simulink model "openMHA_test_ar_filter_gaintable"  (R2020a)
settings: Solver=VariableStepAuto  StartTime=0.0  StopTime=stop_time  RelTol=1e-3
InitFcn:
  | test_ar_filter_gaintable_init
StopFcn:
  | test_ar_filter_gaintable_stop
values from neighbouring files (symbols this model uses):
  c1_a = exp( -1.0/(tau_a * fs) )    [test_FFT_to_gain_init.m]    (also in test_ar_filter_gaintable_init.m; test_ar_filter_init.m; test_db_ar_gaintable_init.m)
  c1_r = exp( -1.0/(tau_r * fs) )    [test_FFT_to_gain_init.m]    (also in test_ar_filter_gaintable_init.m; test_ar_filter_init.m; test_db_ar_gaintable_init.m)
  c2_a = 1.0 - c1_a    [test_FFT_to_gain_init.m]    (also in test_ar_filter_gaintable_init.m; test_ar_filter_init.m; test_db_ar_gaintable_init.m)
  c2_r = 1.0 - c1_r    [test_FFT_to_gain_init.m]    (also in test_ar_filter_gaintable_init.m; test_ar_filter_init.m; test_db_ar_gaintable_init.m)
  table_length = length(gtdata)    [calculate_gaintable.m]    (also in test_FFT_to_gain_init.m; test_ar_filter_gaintable_init.m; test_db_ar_gaintable_init.m; test_db_lookup_gain_fpga_init.m)
  X_high = 93    [test_FFT_to_gain_init.m]    (also in test_ar_filter_gaintable_init.m = 95; test_db_ar_gaintable_init.m; test_db_lookup_gain_fpga_init.m = 95; test_db_lookup_init.m = 95)
libraries: simulink x4, FPGA_Open_Speech_Tools x2, dspsrcs4 x1
settings Model: PacingRate=200  Creator=t96f346  LastModifiedBy=t96f346

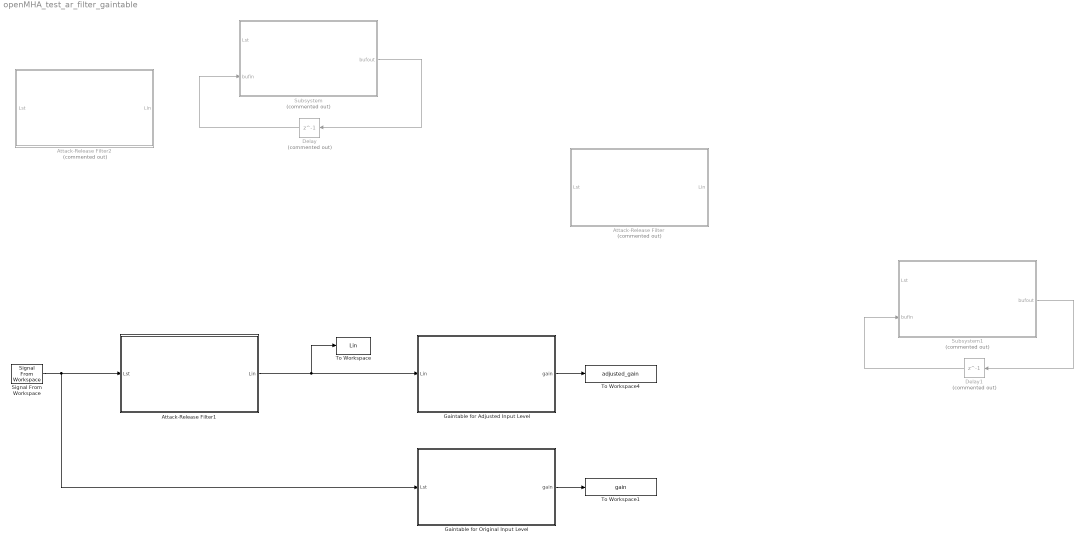
== system openMHA_test_ar_filter_gaintable ==
  Attack-Release Filter : Subsystem  Commented=on
  Attack-Release Filter1 : Subsystem
  Attack-Release Filter2 : Subsystem  Commented=on
  Delay : Delay  Commented=on  DelayLength=1  InitialCondition=65
  Delay1 : Delay  Commented=on  DelayLength=1  InitialCondition=65
  Gaintable for Adjusted Input Level : Subsystem
  Gaintable for Original Input Level : Subsystem
  Signal From Workspace : dspsrcs4/Signal From Workspace  X=Lst  Ts=1  nsamps=1  OutputAfterFinalValue=Setting to zero  ignoreOrWarnInputAndFrameLengths=off  OutputFrames=off
  Subsystem : Subsystem  Commented=on
  Subsystem1 : Subsystem  Commented=on
  To Workspace : ToWorkspace  VariableName=Lin  SampleTime=-1
      settings: Save2DSignal=2-D array (concatenate along first dimension)
  To Workspace1 : ToWorkspace  VariableName=gain  SampleTime=-1
      settings: Save2DSignal=2-D array (concatenate along first dimension)
  To Workspace4 : ToWorkspace  VariableName=adjusted_gain  SampleTime=-1
      settings: Save2DSignal=2-D array (concatenate along first dimension)
  wires:
  Delay/1 -> Subsystem/2(bufin)
  Subsystem/1(bufout) -> Delay/1
  Attack-Release Filter1/1(Lin) -> To Workspace/1, Gaintable for Adjusted Input Level/1(Lin)
  Gaintable for Adjusted Input Level/1(gain) -> To Workspace4/1
  Gaintable for Original Input Level/1(gain) -> To Workspace1/1
  Signal From Workspace/1 -> Attack-Release Filter1/1(Lst), Gaintable for Original Input Level/1(Lst)
  Delay1/1 -> Subsystem1/2(bufin)
  Subsystem1/1(bufout) -> Delay1/1

== system openMHA_test_ar_filter_gaintable/Attack-Release Filter ==
  Lst : Inport
  Delay2 : Delay  DelayLength=1  InitialCondition=65
  Release Filter : Subsystem  TreatAsAtomicUnit=on
  Lin : Outport  VectorParamsAs1DForOutWhenUnconnected=off
  wires:
  Release Filter/1(bufout) -> Lin/1, Delay2/1
  Lst/1 -> Release Filter/1(La)
  Delay2/1 -> Release Filter/2(bufin)

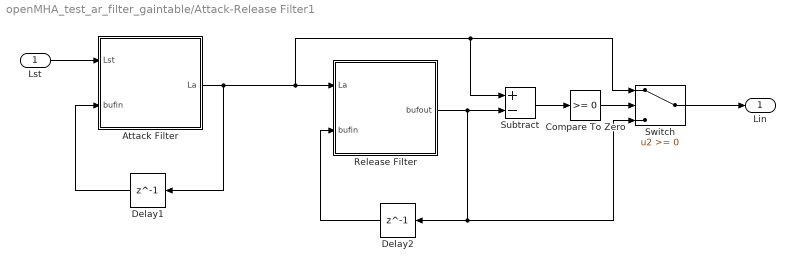
== system openMHA_test_ar_filter_gaintable/Attack-Release Filter1 ==
  Lst : Inport
  Attack Filter : Subsystem  TreatAsAtomicUnit=on
  Compare To Zero : simulink/Logic and Bit Operations/Compare To Zero  relop=>=  OutDataTypeStr=boolean
  Delay1 : Delay  DelayLength=1  InitialCondition=65
  Delay2 : Delay  DelayLength=1  InitialCondition=65
  Release Filter : Subsystem  TreatAsAtomicUnit=on
  Subtract : Sum  Inputs=+-  OutDataTypeStr=Inherit: Same as accumulator
  Switch : Switch
  Lin : Outport  VectorParamsAs1DForOutWhenUnconnected=off
  wires:
  Lst/1 -> Attack Filter/1(Lst)
  Delay2/1 -> Release Filter/2(bufin)
  Delay1/1 -> Attack Filter/2(bufin)
  Release Filter/1(bufout) -> Switch/3, Delay2/1, Subtract/2
  Switch/1 -> Lin/1
  Compare To Zero/1 -> Switch/2
  Attack Filter/1(La) -> Subtract/1, Switch/1, Release Filter/1(La), Delay1/1
  Subtract/1 -> Compare To Zero/1

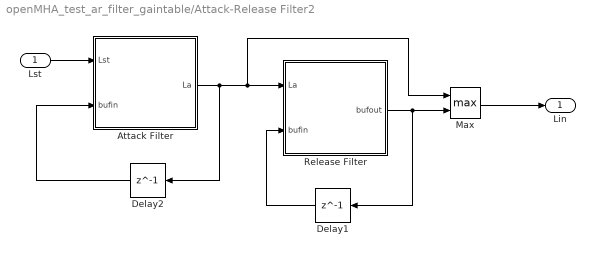
== system openMHA_test_ar_filter_gaintable/Attack-Release Filter2 ==
  Lst : Inport
  Attack Filter : Subsystem  TreatAsAtomicUnit=on
  Delay1 : Delay  DelayLength=1  InitialCondition=65
  Delay2 : Delay  DelayLength=1  InitialCondition=65
  Max : MinMax  Function=max  Inputs=2
  Release Filter : Subsystem  TreatAsAtomicUnit=on
  Lin : Outport  VectorParamsAs1DForOutWhenUnconnected=off
  wires:
  Lst/1 -> Attack Filter/1(Lst)
  Attack Filter/1(La) -> Delay2/1, Max/1, Release Filter/1(La)
  Release Filter/1(bufout) -> Delay1/1, Max/2
  Max/1 -> Lin/1
  Delay2/1 -> Attack Filter/2(bufin)
  Delay1/1 -> Release Filter/2(bufin)

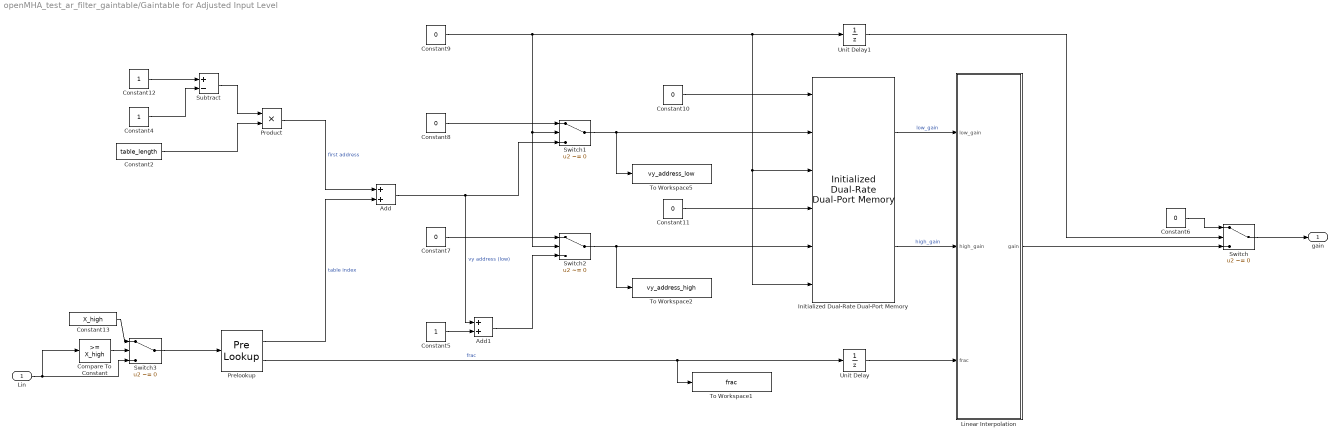
== system openMHA_test_ar_filter_gaintable/Gaintable for Adjusted Input Level ==
  Lin : Inport
  Add : Sum  OutDataTypeStr=uint8
  Add1 : Sum  OutDataTypeStr=uint8
  Compare To Constant : simulink/Logic and Bit Operations/Compare To Constant  relop=>=  const=X_high  OutDataTypeStr=boolean
  Constant10 : Constant  Value=0  OutDataTypeStr=double  SampleTime=-1
  Constant11 : Constant  Value=0  OutDataTypeStr=double  SampleTime=-1
  Constant12 : Constant  OutDataTypeStr=uint8  SampleTime=-1
  Constant13 : Constant  Value=X_high  OutDataTypeStr=fixdt(1,Wbits, Fbits-5)  SampleTime=-1
  Constant2 : Constant  Value=table_length  OutDataTypeStr=uint8  SampleTime=-1
  Constant4 : Constant  OutDataTypeStr=uint8  SampleTime=-1
  Constant5 : Constant  OutDataTypeStr=uint8  SampleTime=-1
  Constant6 : Constant  Value=0  OutDataTypeStr=double  SampleTime=-1
  Constant7 : Constant  Value=0  OutDataTypeStr=uint8  SampleTime=-1
  Constant8 : Constant  Value=0  OutDataTypeStr=uint8  SampleTime=-1
  Constant9 : Constant  Value=0  OutDataTypeStr=boolean  SampleTime=-1
  Initialized Dual-Rate Dual-Port Memory : FPGA_Open_Speech_Tools/Initialized Dual-Rate Dual-Port Memory  ram_size=RAM_size  Table_Init=vy
      settings: SourceProductName=FPGA Open Speech Tools
  Linear Interpolation : Subsystem
  Prelookup : PreLookup  BreakpointsData=input_levels_db  IndexSearchMethod=Evenly spaced points  UseLastBreakpoint=on  DiagnosticForOutOfRangeInput=Error  IndexDataTypeStr=uint8
  Product : Product  OutDataTypeStr=Inherit: Same as first input
  Subtract : Sum  Inputs=+-
  Switch : Switch  Criteria=u2 ~= 0  OutDataTypeStr=double
  Switch1 : Switch  Criteria=u2 ~= 0  OutDataTypeStr=uint8
  Switch2 : Switch  Criteria=u2 ~= 0  OutDataTypeStr=uint8
  Switch3 : Switch  Criteria=u2 ~= 0
  To Workspace1 : ToWorkspace  VariableName=frac  SampleTime=-1
      settings: Save2DSignal=2-D array (concatenate along first dimension)
  To Workspace2 : ToWorkspace  VariableName=vy_address_high  SampleTime=-1
      settings: Save2DSignal=2-D array (concatenate along first dimension)
  To Workspace5 : ToWorkspace  VariableName=vy_address_low  SampleTime=-1
      settings: Save2DSignal=2-D array (concatenate along first dimension)
  Unit Delay : UnitDelay  SampleTime=-1  HasFrameUpgradeWarning=on
  Unit Delay1 : UnitDelay  InitialCondition=1  SampleTime=-1  HasFrameUpgradeWarning=on
  gain : Outport
  wires:
  Constant10/1 -> Initialized Dual-Rate Dual-Port Memory/1
  Unit Delay/1 -> Linear Interpolation/3(frac)
  Unit Delay1/1 -> Switch/2
  Compare To Constant/1 -> Switch3/2
  Switch/1 -> gain/1
  Constant12/1 -> Subtract/1
  Constant6/1 -> Switch/1
  Add/1 -> Switch1/3, Add1/1  "vy address (low)"
  Linear Interpolation/1(gain) -> Switch/3
  Initialized Dual-Rate Dual-Port Memory/2 -> Linear Interpolation/2(high_gain)  "high_gain"
  Switch1/1 -> Initialized Dual-Rate Dual-Port Memory/2, To Workspace5/1
  Constant7/1 -> Switch2/1
  Constant8/1 -> Switch1/1
  Constant5/1 -> Add1/2
  Prelookup/1 -> Add/2  "table index"
  Constant13/1 -> Switch3/1
  Add1/1 -> Switch2/3
  Initialized Dual-Rate Dual-Port Memory/1 -> Linear Interpolation/1(low_gain)  "low_gain"
  Switch2/1 -> Initialized Dual-Rate Dual-Port Memory/5, To Workspace2/1
  Constant4/1 -> Subtract/2
  Constant11/1 -> Initialized Dual-Rate Dual-Port Memory/4
  Prelookup/2 -> To Workspace1/1, Unit Delay/1  "frac"
  Product/1 -> Add/1  "first address"
  Subtract/1 -> Product/1
  Constant9/1 -> Initialized Dual-Rate Dual-Port Memory/3, Initialized Dual-Rate Dual-Port Memory/6, Unit Delay1/1, Switch1/2, Switch2/2
  Lin/1 -> Compare To Constant/1, Switch3/3
  Constant2/1 -> Product/2
  Switch3/1 -> Prelookup/1

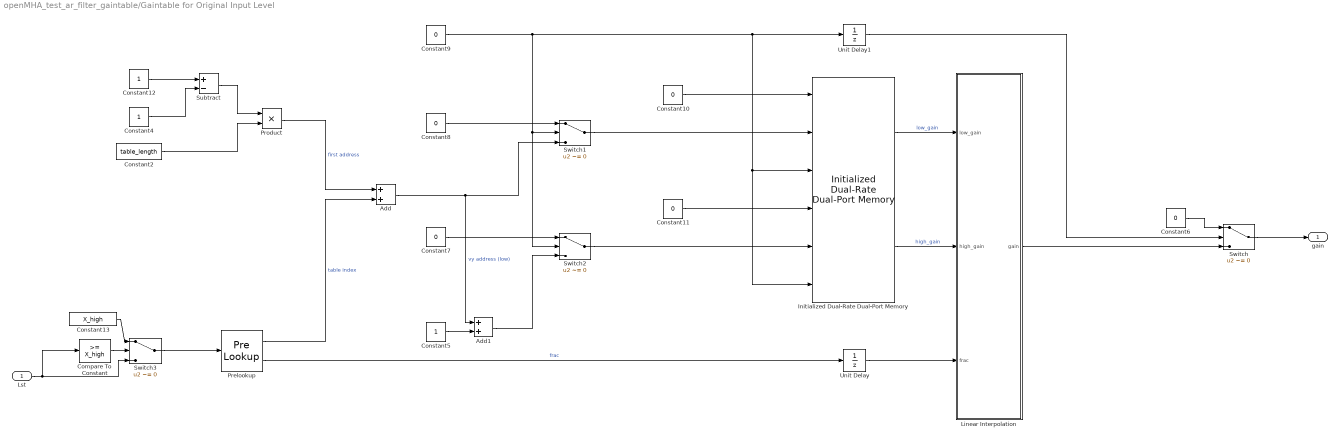
== system openMHA_test_ar_filter_gaintable/Gaintable for Original Input Level ==
  Lst : Inport
  Add : Sum  OutDataTypeStr=uint8
  Add1 : Sum  OutDataTypeStr=uint8
  Compare To Constant : simulink/Logic and Bit Operations/Compare To Constant  relop=>=  const=X_high  OutDataTypeStr=boolean
  Constant10 : Constant  Value=0  OutDataTypeStr=double  SampleTime=-1
  Constant11 : Constant  Value=0  OutDataTypeStr=double  SampleTime=-1
  Constant12 : Constant  OutDataTypeStr=uint8  SampleTime=-1
  Constant13 : Constant  Value=X_high  OutDataTypeStr=fixdt(1,Wbits, Fbits-5)  SampleTime=-1
  Constant2 : Constant  Value=table_length  OutDataTypeStr=uint8  SampleTime=-1
  Constant4 : Constant  OutDataTypeStr=uint8  SampleTime=-1
  Constant5 : Constant  OutDataTypeStr=uint8  SampleTime=-1
  Constant6 : Constant  Value=0  OutDataTypeStr=double  SampleTime=-1
  Constant7 : Constant  Value=0  OutDataTypeStr=uint8  SampleTime=-1
  Constant8 : Constant  Value=0  OutDataTypeStr=uint8  SampleTime=-1
  Constant9 : Constant  Value=0  OutDataTypeStr=boolean  SampleTime=-1
  Initialized Dual-Rate Dual-Port Memory : FPGA_Open_Speech_Tools/Initialized Dual-Rate Dual-Port Memory  ram_size=RAM_size  Table_Init=vy
      settings: SourceProductName=FPGA Open Speech Tools
  Linear Interpolation : Subsystem
  Prelookup : PreLookup  BreakpointsData=input_levels_db  IndexSearchMethod=Evenly spaced points  UseLastBreakpoint=on  DiagnosticForOutOfRangeInput=Error  IndexDataTypeStr=uint8
  Product : Product  OutDataTypeStr=Inherit: Same as first input
  Subtract : Sum  Inputs=+-
  Switch : Switch  Criteria=u2 ~= 0  OutDataTypeStr=double
  Switch1 : Switch  Criteria=u2 ~= 0  OutDataTypeStr=uint8
  Switch2 : Switch  Criteria=u2 ~= 0  OutDataTypeStr=uint8
  Switch3 : Switch  Criteria=u2 ~= 0
  Unit Delay : UnitDelay  SampleTime=-1  HasFrameUpgradeWarning=on
  Unit Delay1 : UnitDelay  InitialCondition=1  SampleTime=-1  HasFrameUpgradeWarning=on
  gain : Outport
  wires:
  Constant10/1 -> Initialized Dual-Rate Dual-Port Memory/1
  Unit Delay/1 -> Linear Interpolation/3(frac)
  Unit Delay1/1 -> Switch/2
  Compare To Constant/1 -> Switch3/2
  Switch/1 -> gain/1
  Constant12/1 -> Subtract/1
  Constant6/1 -> Switch/1
  Add/1 -> Switch1/3, Add1/1  "vy address (low)"
  Linear Interpolation/1(gain) -> Switch/3
  Initialized Dual-Rate Dual-Port Memory/2 -> Linear Interpolation/2(high_gain)  "high_gain"
  Switch1/1 -> Initialized Dual-Rate Dual-Port Memory/2
  Constant7/1 -> Switch2/1
  Constant8/1 -> Switch1/1
  Constant5/1 -> Add1/2
  Prelookup/1 -> Add/2  "table index"
  Constant13/1 -> Switch3/1
  Add1/1 -> Switch2/3
  Initialized Dual-Rate Dual-Port Memory/1 -> Linear Interpolation/1(low_gain)  "low_gain"
  Switch2/1 -> Initialized Dual-Rate Dual-Port Memory/5
  Constant4/1 -> Subtract/2
  Constant11/1 -> Initialized Dual-Rate Dual-Port Memory/4
  Prelookup/2 -> Unit Delay/1  "frac"
  Product/1 -> Add/1  "first address"
  Subtract/1 -> Product/1
  Constant9/1 -> Initialized Dual-Rate Dual-Port Memory/3, Initialized Dual-Rate Dual-Port Memory/6, Unit Delay1/1, Switch1/2, Switch2/2
  Lst/1 -> Compare To Constant/1, Switch3/3
  Constant2/1 -> Product/2
  Switch3/1 -> Prelookup/1

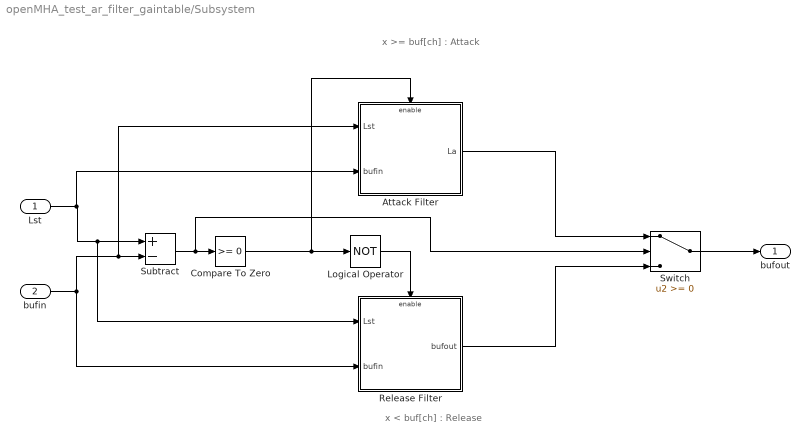
== system openMHA_test_ar_filter_gaintable/Subsystem ==
  note: x < buf[ch] :
      | Release
  note: x >= buf[ch] :
      | Attack
  Lst : Inport
  bufin : Inport  Port=2
  Attack Filter : Subsystem  TreatAsAtomicUnit=on
  Compare To Zero : simulink/Logic and Bit Operations/Compare To Zero  relop=>=  OutDataTypeStr=boolean
  Logical Operator : Logic  Operator=NOT  AllPortsSameDT=off  OutDataTypeStr=boolean
  Release Filter : Subsystem  TreatAsAtomicUnit=on
  Subtract : Sum  Inputs=+-  OutDataTypeStr=Inherit: Same as accumulator
  Switch : Switch
  bufout : Outport  VectorParamsAs1DForOutWhenUnconnected=off
  wires:
  Attack Filter/1(La) -> Switch/1
  Lst/1 -> Attack Filter/2(bufin), Release Filter/1(Lst), Subtract/1
  Subtract/1 -> Switch/2, Compare To Zero/1
  Compare To Zero/1 -> Attack Filter/Enable, Logical Operator/1
  Logical Operator/1 -> Release Filter/Enable
  bufin/1 -> Release Filter/2(bufin), Attack Filter/1(Lst), Subtract/2
  Switch/1 -> bufout/1
  Release Filter/1(bufout) -> Switch/3

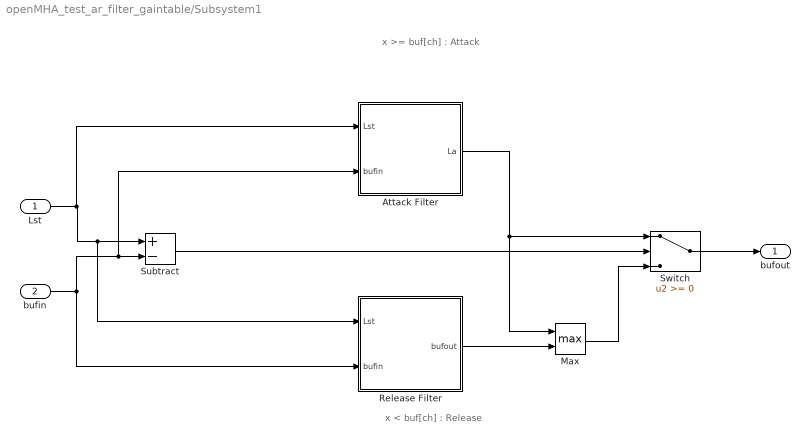
== system openMHA_test_ar_filter_gaintable/Subsystem1 ==
  note: x < buf[ch] :
      | Release
  note: x >= buf[ch] :
      | Attack
  Lst : Inport
  bufin : Inport  Port=2
  Attack Filter : Subsystem  TreatAsAtomicUnit=on
  Max : MinMax  Function=max  Inputs=2
  Release Filter : Subsystem  TreatAsAtomicUnit=on
  Subtract : Sum  Inputs=+-  OutDataTypeStr=Inherit: Same as accumulator
  Switch : Switch
  bufout : Outport  VectorParamsAs1DForOutWhenUnconnected=off
  wires:
  Attack Filter/1(La) -> Max/1, Switch/1
  Lst/1 -> Attack Filter/1(Lst), Release Filter/1(Lst), Subtract/1
  Subtract/1 -> Switch/2
  bufin/1 -> Release Filter/2(bufin), Attack Filter/2(bufin), Subtract/2
  Switch/1 -> bufout/1
  Release Filter/1(bufout) -> Max/2
  Max/1 -> Switch/3

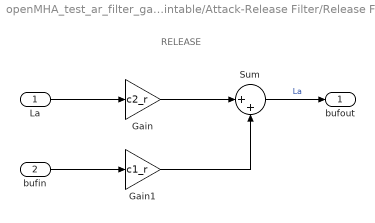
== system openMHA_test_ar_filter_gaintable/Attack-Release Filter/Release Filter ==
  note: RELEASE
  La : Inport
  bufin : Inport  Port=2
  Gain : Gain  Gain=c2_r
  Gain1 : Gain  Gain=c1_r
  Sum : Sum  Inputs=|++
  bufout : Outport  InitialOutput=0  VectorParamsAs1DForOutWhenUnconnected=off
  wires:
  Sum/1 -> bufout/1  "La"
  Gain/1 -> Sum/1
  Gain1/1 -> Sum/2
  bufin/1 -> Gain1/1
  La/1 -> Gain/1

== system openMHA_test_ar_filter_gaintable/Attack-Release Filter1/Attack Filter ==
  note: ATTACK
  Lst : Inport
  bufin : Inport  Port=2
  Gain : Gain  Gain=c2_a
  Gain1 : Gain  Gain=c1_a
  Sum : Sum  Inputs=|++
  La : Outport  InitialOutput=0  VectorParamsAs1DForOutWhenUnconnected=off
  wires:
  Lst/1 -> Gain/1
  Gain/1 -> Sum/1
  Sum/1 -> La/1  "La"
  bufin/1 -> Gain1/1
  Gain1/1 -> Sum/2

== system openMHA_test_ar_filter_gaintable/Attack-Release Filter1/Release Filter ==
  note: RELEASE
  La : Inport
  bufin : Inport  Port=2
  Gain : Gain  Gain=c2_r
  Gain1 : Gain  Gain=c1_r
  Sum : Sum  Inputs=|++
  bufout : Outport  InitialOutput=0  VectorParamsAs1DForOutWhenUnconnected=off
  wires:
  Sum/1 -> bufout/1  "La"
  Gain/1 -> Sum/1
  Gain1/1 -> Sum/2
  bufin/1 -> Gain1/1
  La/1 -> Gain/1

== system openMHA_test_ar_filter_gaintable/Attack-Release Filter2/Attack Filter ==
  note: ATTACK
  Lst : Inport
  bufin : Inport  Port=2
  Gain : Gain  Gain=c2_a
  Gain1 : Gain  Gain=c1_a
  Sum : Sum  Inputs=|++
  La : Outport  InitialOutput=0  VectorParamsAs1DForOutWhenUnconnected=off
  wires:
  Lst/1 -> Gain/1
  Gain/1 -> Sum/1
  Sum/1 -> La/1  "La"
  bufin/1 -> Gain1/1
  Gain1/1 -> Sum/2

== system openMHA_test_ar_filter_gaintable/Attack-Release Filter2/Release Filter ==
  note: RELEASE
  La : Inport
  bufin : Inport  Port=2
  Gain : Gain  Gain=c2_r
  Gain1 : Gain  Gain=c1_r
  Sum : Sum  Inputs=|++
  bufout : Outport  InitialOutput=0  VectorParamsAs1DForOutWhenUnconnected=off
  wires:
  Sum/1 -> bufout/1  "La"
  Gain/1 -> Sum/1
  Gain1/1 -> Sum/2
  bufin/1 -> Gain1/1
  La/1 -> Gain/1

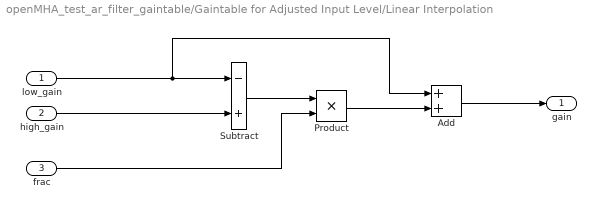
== system openMHA_test_ar_filter_gaintable/Gaintable for Adjusted Input Level/Linear Interpolation ==
  low_gain : Inport
  high_gain : Inport  Port=2
  frac : Inport  Port=3
  Add : Sum
  Product : Product
  Subtract : Sum  Inputs=-+
  gain : Outport
  wires:
  high_gain/1 -> Subtract/2
  low_gain/1 -> Add/1, Subtract/1
  Subtract/1 -> Product/1
  frac/1 -> Product/2
  Product/1 -> Add/2
  Add/1 -> gain/1

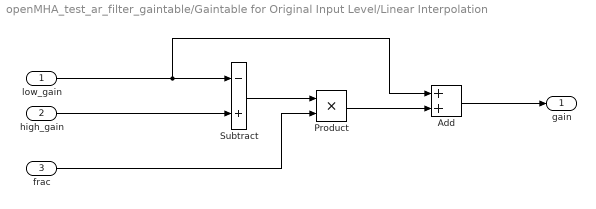
== system openMHA_test_ar_filter_gaintable/Gaintable for Original Input Level/Linear Interpolation ==
  low_gain : Inport
  high_gain : Inport  Port=2
  frac : Inport  Port=3
  Add : Sum
  Product : Product
  Subtract : Sum  Inputs=-+
  gain : Outport
  wires:
  high_gain/1 -> Subtract/2
  low_gain/1 -> Add/1, Subtract/1
  Subtract/1 -> Product/1
  frac/1 -> Product/2
  Product/1 -> Add/2
  Add/1 -> gain/1

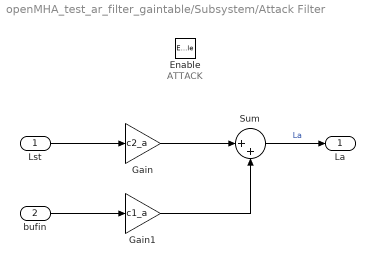
== system openMHA_test_ar_filter_gaintable/Subsystem/Attack Filter ==
  note: ATTACK
  Lst : Inport
  bufin : Inport  Port=2
  Enable : EnablePort
  Gain : Gain  Gain=c2_a
  Gain1 : Gain  Gain=c1_a
  Sum : Sum  Inputs=|++
  La : Outport  InitialOutput=0  VectorParamsAs1DForOutWhenUnconnected=off
  wires:
  Lst/1 -> Gain/1
  Gain/1 -> Sum/1
  Sum/1 -> La/1  "La"
  bufin/1 -> Gain1/1
  Gain1/1 -> Sum/2

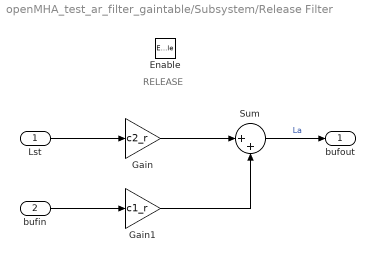
== system openMHA_test_ar_filter_gaintable/Subsystem/Release Filter ==
  note: RELEASE
  Lst : Inport
  bufin : Inport  Port=2
  Enable : EnablePort
  Gain : Gain  Gain=c2_r
  Gain1 : Gain  Gain=c1_r
  Sum : Sum  Inputs=|++
  bufout : Outport  InitialOutput=0  VectorParamsAs1DForOutWhenUnconnected=off
  wires:
  Sum/1 -> bufout/1  "La"
  Gain/1 -> Sum/1
  Gain1/1 -> Sum/2
  bufin/1 -> Gain1/1
  Lst/1 -> Gain/1

== system openMHA_test_ar_filter_gaintable/Subsystem1/Attack Filter ==
  note: ATTACK
  Lst : Inport
  bufin : Inport  Port=2
  Gain : Gain  Gain=c2_a
  Gain1 : Gain  Gain=c1_a
  Sum : Sum  Inputs=|++
  La : Outport  InitialOutput=0  VectorParamsAs1DForOutWhenUnconnected=off
  wires:
  Lst/1 -> Gain/1
  Gain/1 -> Sum/1
  Sum/1 -> La/1  "La"
  bufin/1 -> Gain1/1
  Gain1/1 -> Sum/2

== system openMHA_test_ar_filter_gaintable/Subsystem1/Release Filter ==
  note: RELEASE
  Lst : Inport
  bufin : Inport  Port=2
  Gain : Gain  Gain=c2_r
  Gain1 : Gain  Gain=c1_r
  Sum : Sum  Inputs=|++
  bufout : Outport  InitialOutput=0  VectorParamsAs1DForOutWhenUnconnected=off
  wires:
  Sum/1 -> bufout/1  "La"
  Gain/1 -> Sum/1
  Gain1/1 -> Sum/2
  bufin/1 -> Gain1/1
  Lst/1 -> Gain/1
